simulink model "VCU10"  (R2021b)
settings: Solver=FixedStepDiscrete  StartTime=0.0  StopTime=10.0  FixedStep=0.01  RelTol=1e-3
values from neighbouring files (symbols this model uses):
  F = 0.0    [VCU10DB.sldd]
  FSEC_ESP_EMERGENCY_PRESSURE_MPA = 8.0    [VCU10DB.sldd]
  T = 1.0    [VCU10DB.sldd]
libraries: simulink x148, hdlsllib x90
(part 3 of 4)

== system VCU10/EPS/EPS_ReceiveMsg/EPS_Send_Msg2 ==
  canb_epssendmsg2 : Inport
  Add1 : Sum  Inputs=-++
  Add2 : Sum
  Add5 : Sum  Inputs=-++
  Bit Shift1 : hdlsllib/Logic and Bit Operations/Bit Shift  mode=Shift Left Logical  N=8
  Bus Creator : BusCreator  Inputs=5
  Constant1 : Constant  Value=1024  OutDataTypeStr=uint16
  Constant2 : Constant  Value=1024  OutDataTypeStr=uint16
  Data Type Conversion1 : DataTypeConversion  OutDataTypeStr=double
  Data Type Conversion{3..6,8,10} (6 alike) : DataTypeConversion  OutDataTypeStr=uint16
  Data Type Conversion2 : DataTypeConversion  OutDataTypeStr=double
  Demux : Demux  Outputs=8
  Gain1 : Gain  Gain=256
  Gain2 : Gain  Gain=256
  canb_epssendmsg2signal : Outport
  wires:
  canb_epssendmsg2/1 -> Demux/1
  Bus Creator/1 -> canb_epssendmsg2signal/1
  Demux/1 -> Bus Creator/1  "eps_mode"
  Data Type Conversion2/1 -> Bus Creator/4  "actual_angle"
  Data Type Conversion6/1 -> Gain2/1
  Data Type Conversion5/1 -> Add1/3
  Constant1/1 -> Add1/1
  Gain2/1 -> Add1/2
  Add1/1 -> Data Type Conversion2/1
  Data Type Conversion1/1 -> Bus Creator/3  "received_angle"
  Data Type Conversion8/1 -> Gain1/1
  Data Type Conversion10/1 -> Add5/3
  Constant2/1 -> Add5/1
  Gain1/1 -> Add5/2
  Add5/1 -> Data Type Conversion1/1
  Add2/1 -> Bus Creator/2  "received_command_number"
  Bit Shift1/1 -> Add2/1
  Data Type Conversion3/1 -> Bit Shift1/1
  Data Type Conversion4/1 -> Add2/2
  Demux/2 -> Data Type Conversion3/1  "eps_send_cound"
  Demux/3 -> Data Type Conversion4/1
  Demux/4 -> Data Type Conversion8/1
  Demux/5 -> Data Type Conversion10/1
  Demux/6 -> Data Type Conversion6/1
  Demux/7 -> Data Type Conversion5/1
  Demux/8 -> Bus Creator/5  "eps_send_cound"

== system VCU10/EPS/EPS_TransmitMsg/Subsystem2 ==
  eps_wheel_angle : Inport
  Add1 : Sum
  Constant1 : Constant  Value=1024  OutDataTypeStr=double
  Data Type Conversion4 : DataTypeConversion  OutDataTypeStr=double
  Data Type Conversion5 : DataTypeConversion  OutDataTypeStr=uint32
  Gain1 : Gain  Gain=5
  ipc_cmdangle : Outport
  wires:
  Constant1/1 -> Add1/1
  Add1/1 -> Data Type Conversion5/1
  Data Type Conversion4/1 -> Gain1/1
  Gain1/1 -> Add1/2
  eps_wheel_angle/1 -> Data Type Conversion4/1
  Data Type Conversion5/1 -> ipc_cmdangle/1

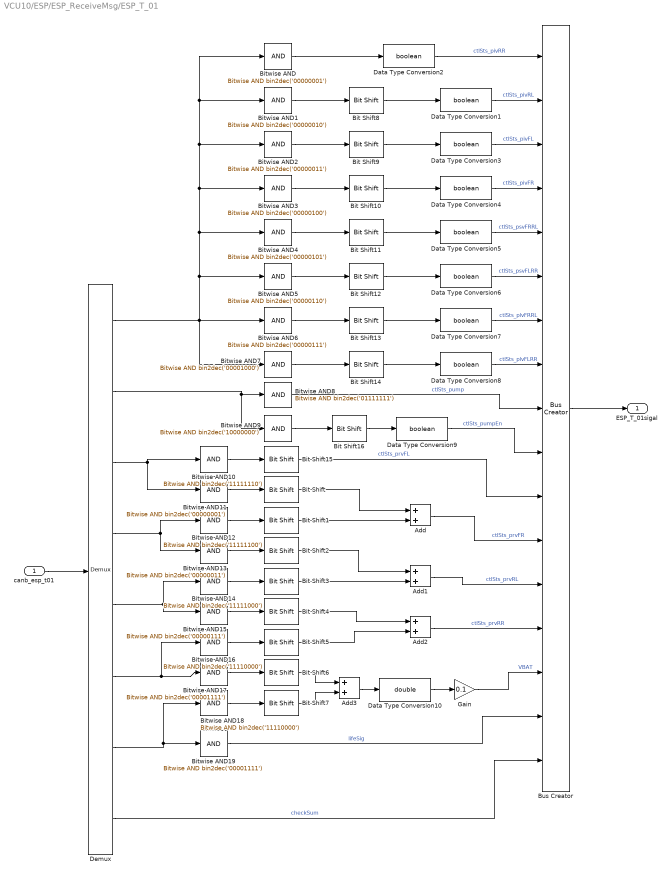
== system VCU10/ESP/ESP_ReceiveMsg/ESP_T_01 ==
  canb_esp_t01 : Inport
  Add{,1..3} (4 alike) : Sum
  Bit Shift : hdlsllib/Logic and Bit Operations/Bit Shift  mode=Shift Left Logical  N=6
  Bit Shift1 : hdlsllib/Logic and Bit Operations/Bit Shift  mode=Shift Right Logical  N=2
  Bit Shift10 : hdlsllib/Logic and Bit Operations/Bit Shift  mode=Shift Right Logical  N=3
  Bit Shift11 : hdlsllib/Logic and Bit Operations/Bit Shift  mode=Shift Right Logical  N=4
  Bit Shift12 : hdlsllib/Logic and Bit Operations/Bit Shift  mode=Shift Right Logical  N=5
  Bit Shift13 : hdlsllib/Logic and Bit Operations/Bit Shift  mode=Shift Right Logical  N=6
  Bit Shift14 : hdlsllib/Logic and Bit Operations/Bit Shift  mode=Shift Right Logical  N=7
  Bit Shift15 : hdlsllib/Logic and Bit Operations/Bit Shift  mode=Shift Right Logical  N=1
  Bit Shift16 : hdlsllib/Logic and Bit Operations/Bit Shift  mode=Shift Right Logical  N=7
  Bit Shift2 : hdlsllib/Logic and Bit Operations/Bit Shift  mode=Shift Left Logical  N=5
  Bit Shift3 : hdlsllib/Logic and Bit Operations/Bit Shift  mode=Shift Right Logical  N=3
  Bit Shift4 : hdlsllib/Logic and Bit Operations/Bit Shift  mode=Shift Left Logical  N=4
  Bit Shift5 : hdlsllib/Logic and Bit Operations/Bit Shift  mode=Shift Right Logical  N=4
  Bit Shift6 : hdlsllib/Logic and Bit Operations/Bit Shift  mode=Shift Left Logical  N=4
  Bit Shift7 : hdlsllib/Logic and Bit Operations/Bit Shift  mode=Shift Right Logical  N=4
  Bit Shift8 : hdlsllib/Logic and Bit Operations/Bit Shift  mode=Shift Right Logical  N=1
  Bit Shift9 : hdlsllib/Logic and Bit Operations/Bit Shift  mode=Shift Right Logical  N=2
  Bitwise AND : simulink/Logic and Bit Operations/Bitwise Operator  logicop=AND  UseBitMask=on  BitMask=bin2dec('00000001')  BitMaskRealWorld=Stored Integer
  Bitwise AND1 : simulink/Logic and Bit Operations/Bitwise Operator  logicop=AND  UseBitMask=on  BitMask=bin2dec('00000010')  BitMaskRealWorld=Stored Integer
  Bitwise AND10 : simulink/Logic and Bit Operations/Bitwise Operator  logicop=AND  UseBitMask=on  BitMask=bin2dec('11111110')  BitMaskRealWorld=Stored Integer
  Bitwise AND11 : simulink/Logic and Bit Operations/Bitwise Operator  logicop=AND  UseBitMask=on  BitMask=bin2dec('00000001')  BitMaskRealWorld=Stored Integer
  Bitwise AND12 : simulink/Logic and Bit Operations/Bitwise Operator  logicop=AND  UseBitMask=on  BitMask=bin2dec('11111100')  BitMaskRealWorld=Stored Integer
  Bitwise AND13 : simulink/Logic and Bit Operations/Bitwise Operator  logicop=AND  UseBitMask=on  BitMask=bin2dec('00000011')  BitMaskRealWorld=Stored Integer
  Bitwise AND14 : simulink/Logic and Bit Operations/Bitwise Operator  logicop=AND  UseBitMask=on  BitMask=bin2dec('11111000')  BitMaskRealWorld=Stored Integer
  Bitwise AND15 : simulink/Logic and Bit Operations/Bitwise Operator  logicop=AND  UseBitMask=on  BitMask=bin2dec('00000111')  BitMaskRealWorld=Stored Integer
  Bitwise AND16 : simulink/Logic and Bit Operations/Bitwise Operator  logicop=AND  UseBitMask=on  BitMask=bin2dec('11110000')  BitMaskRealWorld=Stored Integer
  Bitwise AND17 : simulink/Logic and Bit Operations/Bitwise Operator  logicop=AND  UseBitMask=on  BitMask=bin2dec('00001111')  BitMaskRealWorld=Stored Integer
  Bitwise AND18 : simulink/Logic and Bit Operations/Bitwise Operator  logicop=AND  UseBitMask=on  BitMask=bin2dec('11110000')  BitMaskRealWorld=Stored Integer
  Bitwise AND19 : simulink/Logic and Bit Operations/Bitwise Operator  logicop=AND  UseBitMask=on  BitMask=bin2dec('00001111')  BitMaskRealWorld=Stored Integer
  Bitwise AND2 : simulink/Logic and Bit Operations/Bitwise Operator  logicop=AND  UseBitMask=on  BitMask=bin2dec('00000011')  BitMaskRealWorld=Stored Integer
  Bitwise AND3 : simulink/Logic and Bit Operations/Bitwise Operator  logicop=AND  UseBitMask=on  BitMask=bin2dec('00000100')  BitMaskRealWorld=Stored Integer
  Bitwise AND4 : simulink/Logic and Bit Operations/Bitwise Operator  logicop=AND  UseBitMask=on  BitMask=bin2dec('00000101')  BitMaskRealWorld=Stored Integer
  Bitwise AND5 : simulink/Logic and Bit Operations/Bitwise Operator  logicop=AND  UseBitMask=on  BitMask=bin2dec('00000110')  BitMaskRealWorld=Stored Integer
  Bitwise AND6 : simulink/Logic and Bit Operations/Bitwise Operator  logicop=AND  UseBitMask=on  BitMask=bin2dec('00000111')  BitMaskRealWorld=Stored Integer
  Bitwise AND7 : simulink/Logic and Bit Operations/Bitwise Operator  logicop=AND  UseBitMask=on  BitMask=bin2dec('00001000')  BitMaskRealWorld=Stored Integer
  Bitwise AND8 : simulink/Logic and Bit Operations/Bitwise Operator  logicop=AND  UseBitMask=on  BitMask=bin2dec('01111111')  BitMaskRealWorld=Stored Integer
  Bitwise AND9 : simulink/Logic and Bit Operations/Bitwise Operator  logicop=AND  UseBitMask=on  BitMask=bin2dec('10000000')  BitMaskRealWorld=Stored Integer
  Bus Creator : BusCreator  Inputs=17
  Data Type Conversion{1..9} (9 alike) : DataTypeConversion  OutDataTypeStr=boolean
  Data Type Conversion10 : DataTypeConversion  OutDataTypeStr=double
  Demux : Demux  Outputs=8
  Gain : Gain  Gain=0.1
  ESP_T_01sigal : Outport
  wires:
  canb_esp_t01/1 -> Demux/1
  Bus Creator/1 -> ESP_T_01sigal/1
  Bitwise AND/1 -> Data Type Conversion2/1
  Demux/1 -> Bitwise AND/1, Bitwise AND1/1, Bitwise AND2/1, Bitwise AND3/1, Bitwise AND4/1, Bitwise AND5/1, Bitwise AND7/1, Bitwise AND6/1
  Demux/2 -> Bitwise AND9/1, Bitwise AND8/1
  Bitwise AND8/1 -> Bus Creator/9  "ctlSts_pump"
  Bitwise AND10/1 -> Bit Shift15/1
  Demux/4 -> Bitwise AND12/1, Bitwise AND13/1
  Demux/3 -> Bitwise AND10/1, Bitwise AND11/1
  Bitwise AND11/1 -> Bit Shift/1
  Bitwise AND12/1 -> Bit Shift1/1
  Bit Shift1/1 -> Add/2
  Bit Shift/1 -> Add/1
  Add/1 -> Bus Creator/12  "ctlSts_prvFR"
  Bitwise AND13/1 -> Bit Shift2/1
  Demux/5 -> Bitwise AND14/1, Bitwise AND15/1
  Bitwise AND14/1 -> Bit Shift3/1
  Bit Shift2/1 -> Add1/1
  Bit Shift3/1 -> Add1/2
  Add1/1 -> Bus Creator/13  "ctlSts_prvRL"
  Bitwise AND15/1 -> Bit Shift4/1
  Demux/6 -> Bitwise AND16/1, Bitwise AND17/1
  Bitwise AND16/1 -> Bit Shift5/1
  Bit Shift4/1 -> Add2/1
  Bit Shift5/1 -> Add2/2
  Add2/1 -> Bus Creator/14  "ctlSts_prvRR"
  Bitwise AND17/1 -> Bit Shift6/1
  Demux/7 -> Bitwise AND18/1, Bitwise AND19/1
  Bitwise AND18/1 -> Bit Shift7/1
  Bit Shift6/1 -> Add3/1
  Bit Shift7/1 -> Add3/2
  Bitwise AND19/1 -> Bus Creator/16  "lifeSig"
  Demux/8 -> Bus Creator/17  "checkSum"
  Bitwise AND1/1 -> Bit Shift8/1
  Bit Shift8/1 -> Data Type Conversion1/1
  Bitwise AND2/1 -> Bit Shift9/1
  Bit Shift9/1 -> Data Type Conversion3/1
  Bitwise AND3/1 -> Bit Shift10/1
  Bitwise AND4/1 -> Bit Shift11/1
  Bitwise AND5/1 -> Bit Shift12/1
  Bitwise AND6/1 -> Bit Shift13/1
  Bitwise AND7/1 -> Bit Shift14/1
  Bit Shift10/1 -> Data Type Conversion4/1
  Bit Shift11/1 -> Data Type Conversion5/1
  Bit Shift12/1 -> Data Type Conversion6/1
  Bit Shift13/1 -> Data Type Conversion7/1
  Bit Shift14/1 -> Data Type Conversion8/1
  Gain/1 -> Bus Creator/15  "VBAT"
  Data Type Conversion2/1 -> Bus Creator/1  "ctlSts_pivRR"
  Data Type Conversion1/1 -> Bus Creator/2  "ctlSts_pivRL"
  Data Type Conversion3/1 -> Bus Creator/3  "ctlSts_pivFL"
  Data Type Conversion4/1 -> Bus Creator/4  "ctlSts_pivFR"
  Data Type Conversion5/1 -> Bus Creator/5  "ctlSts_psvFRRL"
  Data Type Conversion6/1 -> Bus Creator/6  "ctlSts_psvFLRR"
  Data Type Conversion7/1 -> Bus Creator/7  "ctlSts_plvFRRL"
  Data Type Conversion8/1 -> Bus Creator/8  "ctlSts_plvFLRR"
  Bit Shift15/1 -> Bus Creator/11  "ctlSts_prvFL"
  Bitwise AND9/1 -> Bit Shift16/1
  Bit Shift16/1 -> Data Type Conversion9/1
  Data Type Conversion9/1 -> Bus Creator/10  "ctlSts_pumpEn"
  Data Type Conversion10/1 -> Gain/1
  Add3/1 -> Data Type Conversion10/1

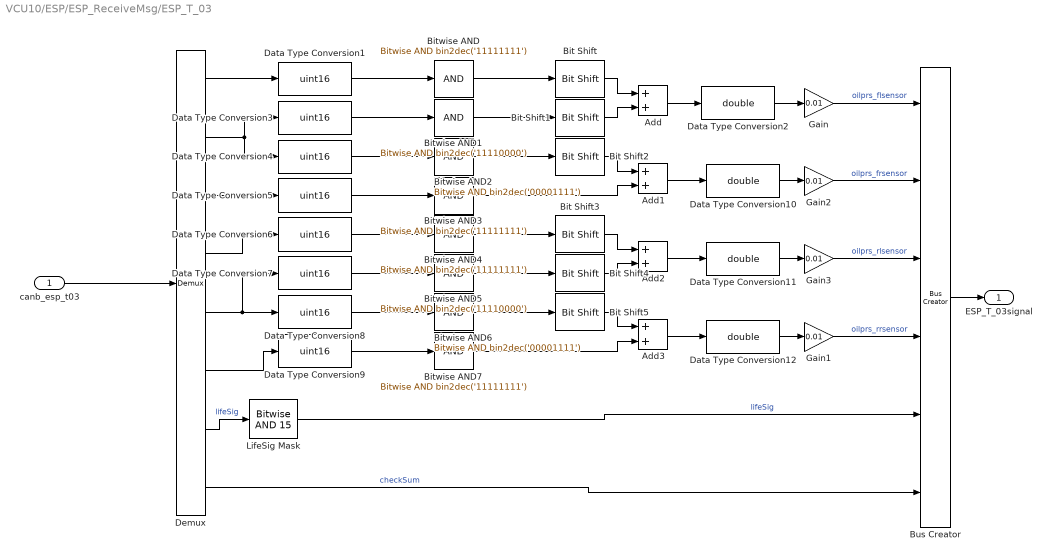
== system VCU10/ESP/ESP_ReceiveMsg/ESP_T_03 ==
  canb_esp_t03 : Inport
  Add{,1..3} (4 alike) : Sum
  Bit Shift : hdlsllib/Logic and Bit Operations/Bit Shift  mode=Shift Left Logical  N=4
  Bit Shift1 : hdlsllib/Logic and Bit Operations/Bit Shift  mode=Shift Right Logical  N=4
  Bit Shift2 : hdlsllib/Logic and Bit Operations/Bit Shift  mode=Shift Left Logical  N=8
  Bit Shift3 : hdlsllib/Logic and Bit Operations/Bit Shift  mode=Shift Left Logical  N=4
  Bit Shift4 : hdlsllib/Logic and Bit Operations/Bit Shift  mode=Shift Right Logical  N=4
  Bit Shift5 : hdlsllib/Logic and Bit Operations/Bit Shift  mode=Shift Left Logical  N=8
  Bitwise AND{,3..4,7} (4 alike) : simulink/Logic and Bit Operations/Bitwise Operator  logicop=AND  UseBitMask=on  BitMask=bin2dec('11111111')  BitMaskRealWorld=Stored Integer
  Bitwise AND1 : simulink/Logic and Bit Operations/Bitwise Operator  logicop=AND  UseBitMask=on  BitMask=bin2dec('11110000')  BitMaskRealWorld=Stored Integer
  Bitwise AND2 : simulink/Logic and Bit Operations/Bitwise Operator  logicop=AND  UseBitMask=on  BitMask=bin2dec('00001111')  BitMaskRealWorld=Stored Integer
  Bitwise AND5 : simulink/Logic and Bit Operations/Bitwise Operator  logicop=AND  UseBitMask=on  BitMask=bin2dec('11110000')  BitMaskRealWorld=Stored Integer
  Bitwise AND6 : simulink/Logic and Bit Operations/Bitwise Operator  logicop=AND  UseBitMask=on  BitMask=bin2dec('00001111')  BitMaskRealWorld=Stored Integer
  Bus Creator : BusCreator  Inputs=6
  Data Type Conversion{1,3..9} (8 alike) : DataTypeConversion  OutDataTypeStr=uint16
  Data Type Conversion{2,10..12} (4 alike) : DataTypeConversion  OutDataTypeStr=double
  Demux : Demux  Outputs=8
  Gain{,1..3} (4 alike) : Gain  Gain=0.01
  LifeSig Mask : simulink/Logic and Bit Operations/Bitwise Operator  logicop=AND  UseBitMask=on  BitMask=15  BitMaskRealWorld=Stored Integer
  ESP_T_03signal : Outport
  wires:
  canb_esp_t03/1 -> Demux/1
  Demux/1 -> Data Type Conversion1/1
  Demux/2 -> Data Type Conversion3/1, Data Type Conversion4/1
  Data Type Conversion1/1 -> Bitwise AND/1
  Data Type Conversion3/1 -> Bitwise AND1/1
  Bitwise AND/1 -> Bit Shift/1
  Bitwise AND1/1 -> Bit Shift1/1
  Bit Shift/1 -> Add/1
  Bit Shift1/1 -> Add/2
  Demux/3 -> Data Type Conversion5/1
  Data Type Conversion4/1 -> Bitwise AND2/1
  Bitwise AND2/1 -> Bit Shift2/1
  Data Type Conversion5/1 -> Bitwise AND3/1
  Bit Shift2/1 -> Add1/1
  Bitwise AND3/1 -> Add1/2
  Data Type Conversion6/1 -> Bitwise AND4/1
  Data Type Conversion7/1 -> Bitwise AND5/1
  Bitwise AND4/1 -> Bit Shift3/1
  Bitwise AND5/1 -> Bit Shift4/1
  Bit Shift3/1 -> Add2/1
  Bit Shift4/1 -> Add2/2
  Data Type Conversion8/1 -> Bitwise AND6/1
  Data Type Conversion9/1 -> Bitwise AND7/1
  Bitwise AND6/1 -> Bit Shift5/1
  Bit Shift5/1 -> Add3/1
  Bitwise AND7/1 -> Add3/2
  Demux/4 -> Data Type Conversion6/1
  Demux/5 -> Data Type Conversion8/1, Data Type Conversion7/1
  Demux/6 -> Data Type Conversion9/1
  Demux/8 -> Bus Creator/6  "checkSum"
  Bus Creator/1 -> ESP_T_03signal/1
  Gain/1 -> Bus Creator/1  "oilprs_flsensor"
  Gain3/1 -> Bus Creator/3  "oilprs_rlsensor"
  Gain2/1 -> Bus Creator/2  "oilprs_frsensor"
  Gain1/1 -> Bus Creator/4  "oilprs_rrsensor"
  Add/1 -> Data Type Conversion2/1
  Data Type Conversion2/1 -> Gain/1
  Add1/1 -> Data Type Conversion10/1
  Data Type Conversion10/1 -> Gain2/1
  Add2/1 -> Data Type Conversion11/1
  Data Type Conversion11/1 -> Gain3/1
  Add3/1 -> Data Type Conversion12/1
  Data Type Conversion12/1 -> Gain1/1
  Demux/7 -> LifeSig Mask/1  "lifeSig"
  LifeSig Mask/1 -> Bus Creator/5  "lifeSig"

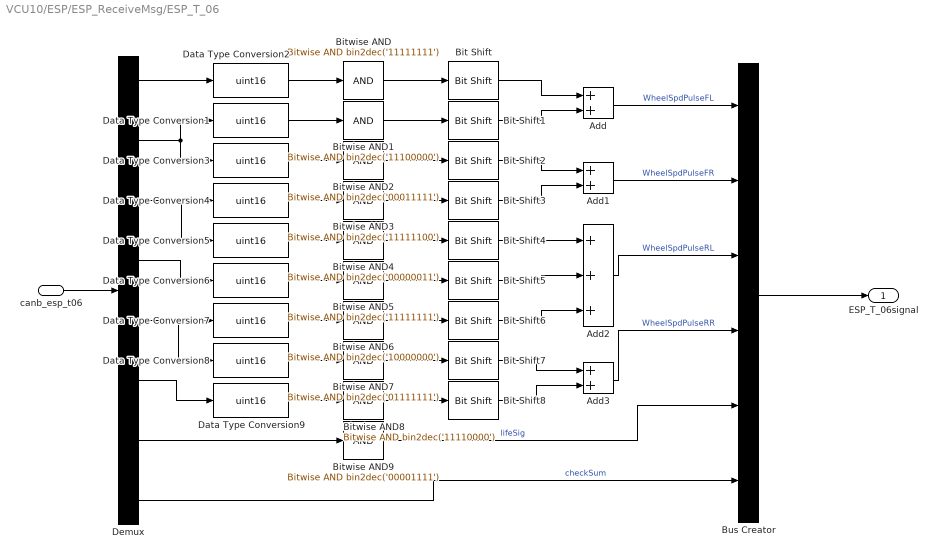
== system VCU10/ESP/ESP_ReceiveMsg/ESP_T_06 ==
  canb_esp_t06 : Inport
  Add : Sum
  Add1 : Sum
  Add2 : Sum  Inputs=+++
  Add3 : Sum
  Bit Shift : hdlsllib/Logic and Bit Operations/Bit Shift  mode=Shift Left Logical  N=3
  Bit Shift1 : hdlsllib/Logic and Bit Operations/Bit Shift  mode=Shift Right Logical  N=5
  Bit Shift2 : hdlsllib/Logic and Bit Operations/Bit Shift  mode=Shift Left Logical  N=6
  Bit Shift3 : hdlsllib/Logic and Bit Operations/Bit Shift  mode=Shift Right Logical  N=2
  Bit Shift4 : hdlsllib/Logic and Bit Operations/Bit Shift  mode=Shift Left Logical  N=9
  Bit Shift5 : hdlsllib/Logic and Bit Operations/Bit Shift  mode=Shift Left Logical  N=1
  Bit Shift6 : hdlsllib/Logic and Bit Operations/Bit Shift  mode=Shift Right Logical  N=7
  Bit Shift7 : hdlsllib/Logic and Bit Operations/Bit Shift  mode=Shift Left Logical  N=4
  Bit Shift8 : hdlsllib/Logic and Bit Operations/Bit Shift  mode=Shift Right Logical  N=4
  Bitwise AND : simulink/Logic and Bit Operations/Bitwise Operator  logicop=AND  UseBitMask=on  BitMask=bin2dec('11111111')  BitMaskRealWorld=Stored Integer
  Bitwise AND1 : simulink/Logic and Bit Operations/Bitwise Operator  logicop=AND  UseBitMask=on  BitMask=bin2dec('11100000')  BitMaskRealWorld=Stored Integer
  Bitwise AND2 : simulink/Logic and Bit Operations/Bitwise Operator  logicop=AND  UseBitMask=on  BitMask=bin2dec('00011111')  BitMaskRealWorld=Stored Integer
  Bitwise AND3 : simulink/Logic and Bit Operations/Bitwise Operator  logicop=AND  UseBitMask=on  BitMask=bin2dec('11111100')  BitMaskRealWorld=Stored Integer
  Bitwise AND4 : simulink/Logic and Bit Operations/Bitwise Operator  logicop=AND  UseBitMask=on  BitMask=bin2dec('00000011')  BitMaskRealWorld=Stored Integer
  Bitwise AND5 : simulink/Logic and Bit Operations/Bitwise Operator  logicop=AND  UseBitMask=on  BitMask=bin2dec('11111111')  BitMaskRealWorld=Stored Integer
  Bitwise AND6 : simulink/Logic and Bit Operations/Bitwise Operator  logicop=AND  UseBitMask=on  BitMask=bin2dec('10000000')  BitMaskRealWorld=Stored Integer
  Bitwise AND7 : simulink/Logic and Bit Operations/Bitwise Operator  logicop=AND  UseBitMask=on  BitMask=bin2dec('01111111')  BitMaskRealWorld=Stored Integer
  Bitwise AND8 : simulink/Logic and Bit Operations/Bitwise Operator  logicop=AND  UseBitMask=on  BitMask=bin2dec('11110000')  BitMaskRealWorld=Stored Integer
  Bitwise AND9 : simulink/Logic and Bit Operations/Bitwise Operator  logicop=AND  UseBitMask=on  BitMask=bin2dec('00001111')  BitMaskRealWorld=Stored Integer
  Bus Creator : BusCreator  Inputs=6
  Data Type Conversion{1..9} (9 alike) : DataTypeConversion  OutDataTypeStr=uint16
  Demux : Demux  Outputs=8
  ESP_T_06signal : Outport
  wires:
  canb_esp_t06/1 -> Demux/1
  Demux/1 -> Data Type Conversion2/1
  Data Type Conversion2/1 -> Bitwise AND/1
  Bitwise AND/1 -> Bit Shift/1
  Data Type Conversion1/1 -> Bitwise AND1/1
  Bitwise AND1/1 -> Bit Shift1/1
  Add/1 -> Bus Creator/1  "WheelSpdPulseFL"
  Bus Creator/1 -> ESP_T_06signal/1
  Demux/2 -> Data Type Conversion3/1, Data Type Conversion1/1
  Data Type Conversion3/1 -> Bitwise AND2/1
  Bitwise AND2/1 -> Bit Shift2/1
  Demux/3 -> Data Type Conversion5/1, Data Type Conversion4/1
  Data Type Conversion4/1 -> Bitwise AND3/1
  Bitwise AND3/1 -> Bit Shift3/1
  Add1/1 -> Bus Creator/2  "WheelSpdPulseFR"
  Bit Shift2/1 -> Add1/1
  Bit Shift3/1 -> Add1/2
  Bit Shift/1 -> Add/1
  Bit Shift1/1 -> Add/2
  Data Type Conversion5/1 -> Bitwise AND4/1
  Bitwise AND4/1 -> Bit Shift4/1
  Demux/4 -> Data Type Conversion6/1
  Data Type Conversion6/1 -> Bitwise AND5/1
  Bitwise AND5/1 -> Bit Shift5/1
  Data Type Conversion7/1 -> Bitwise AND6/1
  Bitwise AND6/1 -> Bit Shift6/1
  Bit Shift4/1 -> Add2/1
  Bit Shift5/1 -> Add2/2
  Bit Shift6/1 -> Add2/3
  Add2/1 -> Bus Creator/3  "WheelSpdPulseRL"
  Demux/5 -> Data Type Conversion8/1, Data Type Conversion7/1
  Data Type Conversion8/1 -> Bitwise AND7/1
  Bitwise AND7/1 -> Bit Shift7/1
  Demux/6 -> Data Type Conversion9/1
  Data Type Conversion9/1 -> Bitwise AND8/1
  Bitwise AND8/1 -> Bit Shift8/1
  Bit Shift7/1 -> Add3/1
  Bit Shift8/1 -> Add3/2
  Add3/1 -> Bus Creator/4  "WheelSpdPulseRR"
  Demux/7 -> Bitwise AND9/1
  Demux/8 -> Bus Creator/6  "checkSum"
  Bitwise AND9/1 -> Bus Creator/5  "lifeSig"

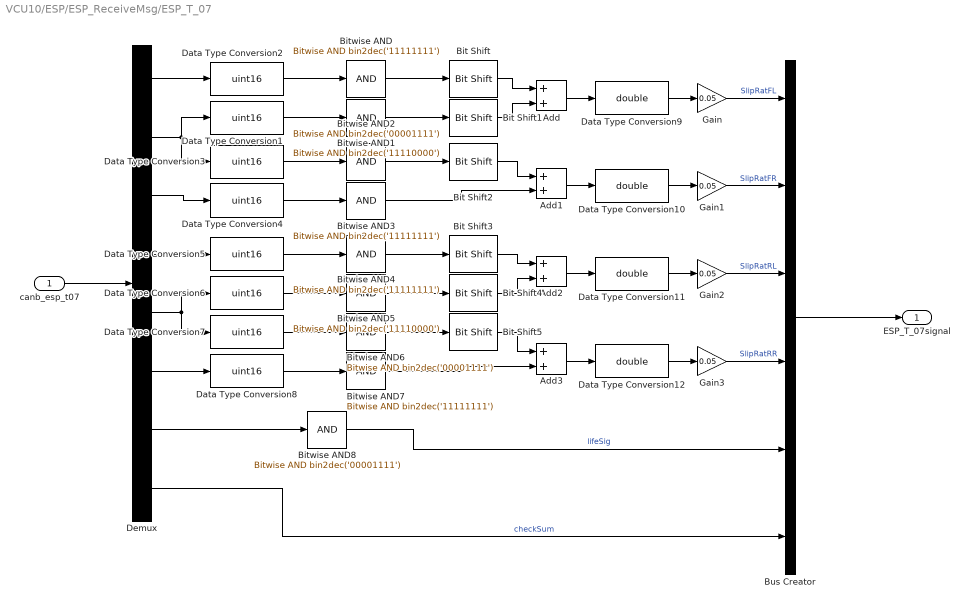
== system VCU10/ESP/ESP_ReceiveMsg/ESP_T_07 ==
  canb_esp_t07 : Inport
  Add{,1..3} (4 alike) : Sum
  Bit Shift : hdlsllib/Logic and Bit Operations/Bit Shift  mode=Shift Left Logical  N=4
  Bit Shift1 : hdlsllib/Logic and Bit Operations/Bit Shift  mode=Shift Right Logical  N=4
  Bit Shift2 : hdlsllib/Logic and Bit Operations/Bit Shift  mode=Shift Left Logical  N=8
  Bit Shift3 : hdlsllib/Logic and Bit Operations/Bit Shift  mode=Shift Left Logical  N=4
  Bit Shift4 : hdlsllib/Logic and Bit Operations/Bit Shift  mode=Shift Right Logical  N=4
  Bit Shift5 : hdlsllib/Logic and Bit Operations/Bit Shift  mode=Shift Left Logical  N=8
  Bitwise AND{,3..4,7} (4 alike) : simulink/Logic and Bit Operations/Bitwise Operator  logicop=AND  UseBitMask=on  BitMask=bin2dec('11111111')  BitMaskRealWorld=Stored Integer
  Bitwise AND1 : simulink/Logic and Bit Operations/Bitwise Operator  logicop=AND  UseBitMask=on  BitMask=bin2dec('11110000')  BitMaskRealWorld=Stored Integer
  Bitwise AND2 : simulink/Logic and Bit Operations/Bitwise Operator  logicop=AND  UseBitMask=on  BitMask=bin2dec('00001111')  BitMaskRealWorld=Stored Integer
  Bitwise AND5 : simulink/Logic and Bit Operations/Bitwise Operator  logicop=AND  UseBitMask=on  BitMask=bin2dec('11110000')  BitMaskRealWorld=Stored Integer
  Bitwise AND6 : simulink/Logic and Bit Operations/Bitwise Operator  logicop=AND  UseBitMask=on  BitMask=bin2dec('00001111')  BitMaskRealWorld=Stored Integer
  Bitwise AND8 : simulink/Logic and Bit Operations/Bitwise Operator  logicop=AND  UseBitMask=on  BitMask=bin2dec('00001111')  BitMaskRealWorld=Stored Integer
  Bus Creator : BusCreator  Inputs=6
  Data Type Conversion{1..8} (8 alike) : DataTypeConversion  OutDataTypeStr=uint16
  Data Type Conversion{9..12} (4 alike) : DataTypeConversion  OutDataTypeStr=double
  Demux : Demux  Outputs=8
  Gain{,1..3} (4 alike) : Gain  Gain=0.05
  ESP_T_07signal : Outport
  wires:
  canb_esp_t07/1 -> Demux/1
  Demux/1 -> Data Type Conversion2/1
  Demux/2 -> Data Type Conversion1/1, Data Type Conversion3/1
  Data Type Conversion1/1 -> Bitwise AND1/1
  Data Type Conversion2/1 -> Bitwise AND/1
  Bitwise AND/1 -> Bit Shift/1
  Bitwise AND1/1 -> Bit Shift1/1
  Bit Shift/1 -> Add/1
  Bit Shift1/1 -> Add/2
  Bus Creator/1 -> ESP_T_07signal/1
  Add/1 -> Data Type Conversion9/1
  Gain/1 -> Bus Creator/1  "SlipRatFL"
  Data Type Conversion3/1 -> Bitwise AND2/1
  Bitwise AND2/1 -> Bit Shift2/1
  Add1/1 -> Data Type Conversion10/1
  Gain1/1 -> Bus Creator/2  "SlipRatFR"
  Bit Shift2/1 -> Add1/1
  Demux/3 -> Data Type Conversion4/1
  Data Type Conversion4/1 -> Bitwise AND3/1
  Bitwise AND3/1 -> Add1/2
  Demux/4 -> Data Type Conversion5/1
  Data Type Conversion5/1 -> Bitwise AND4/1
  Bitwise AND4/1 -> Bit Shift3/1
  Add2/1 -> Data Type Conversion11/1
  Bit Shift3/1 -> Add2/1
  Demux/5 -> Data Type Conversion6/1, Data Type Conversion7/1
  Data Type Conversion6/1 -> Bitwise AND5/1
  Bitwise AND5/1 -> Bit Shift4/1
  Bit Shift4/1 -> Add2/2
  Gain2/1 -> Bus Creator/3  "SlipRatRL"
  Data Type Conversion7/1 -> Bitwise AND6/1
  Bitwise AND6/1 -> Bit Shift5/1
  Demux/6 -> Data Type Conversion8/1
  Data Type Conversion8/1 -> Bitwise AND7/1
  Add3/1 -> Data Type Conversion12/1
  Gain3/1 -> Bus Creator/4  "SlipRatRR"
  Bit Shift5/1 -> Add3/1
  Bitwise AND7/1 -> Add3/2
  Demux/7 -> Bitwise AND8/1
  Demux/8 -> Bus Creator/6  "checkSum"
  Data Type Conversion9/1 -> Gain/1
  Data Type Conversion10/1 -> Gain1/1
  Data Type Conversion11/1 -> Gain2/1
  Data Type Conversion12/1 -> Gain3/1
  Bitwise AND8/1 -> Bus Creator/5  "lifeSig"

== system VCU10/ESP/ESP_ReceiveMsg/Subsystem ==
  lifesig : Inport
  brkmotor_check_system : Stateflow chart  TreatAsAtomicUnit=on
  brkmotor_check : Outport
  wires:
  lifesig/1 -> brkmotor_check_system/1(lifesig)
  brkmotor_check_system/1(brkmotor_check) -> brkmotor_check/1

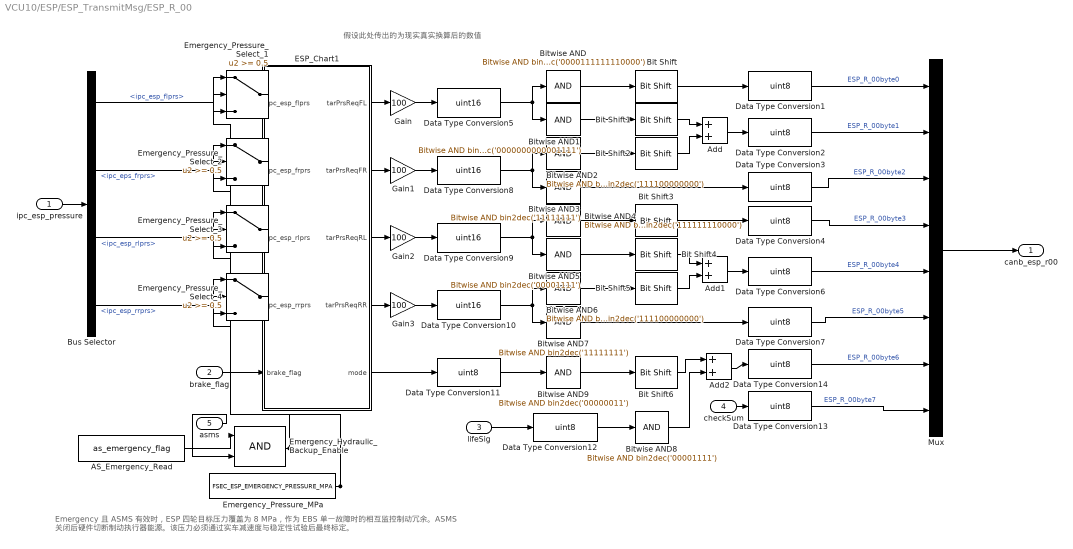
== system VCU10/ESP/ESP_TransmitMsg/ESP_R_00 ==
  note: 假设此处传出的为现实真实换算后的数值
  note: Emergency 且 ASMS 有效时，ESP 四轮目标压力覆盖为 8 MPa，作为 EBS 单一故障时的相互监控制动冗余。ASMS 关闭后硬件切断制动执行器能源。该压力必须通过实车减速度与稳定性试验后最终标定。
  ipc_esp_pressure : Inport
  brake_flag : Inport  Port=2
  lifeSig : Inport  Port=3
  checkSum : Inport  Port=4
  asms : Inport  Port=5  OutDataTypeStr=boolean
  AS_Emergency_Read : DataStoreRead  DataStoreName=as_emergency_flag  IndexOptions=Index vector (dialog)  Indices=1  OutputSizes=1
  Add : Sum
  Add1 : Sum
  Add2 : Sum
  Bit Shift : hdlsllib/Logic and Bit Operations/Bit Shift  mode=Shift Right Logical  N=4
  Bit Shift1 : hdlsllib/Logic and Bit Operations/Bit Shift  mode=Shift Left Logical  N=4
  Bit Shift2 : hdlsllib/Logic and Bit Operations/Bit Shift  mode=Shift Right Logical  N=8
  Bit Shift3 : hdlsllib/Logic and Bit Operations/Bit Shift  mode=Shift Right Logical  N=4
  Bit Shift4 : hdlsllib/Logic and Bit Operations/Bit Shift  mode=Shift Left Logical  N=4
  Bit Shift5 : hdlsllib/Logic and Bit Operations/Bit Shift  mode=Shift Right Logical  N=8
  Bit Shift6 : hdlsllib/Logic and Bit Operations/Bit Shift  mode=Shift Left Logical  N=6
  Bitwise AND : simulink/Logic and Bit Operations/Bitwise Operator  logicop=AND  UseBitMask=on  BitMask=bin2dec('0000111111110000')  BitMaskRealWorld=Stored Integer
  Bitwise AND1 : simulink/Logic and Bit Operations/Bitwise Operator  logicop=AND  UseBitMask=on  BitMask=bin2dec('0000000000001111')  BitMaskRealWorld=Stored Integer
  Bitwise AND2 : simulink/Logic and Bit Operations/Bitwise Operator  logicop=AND  UseBitMask=on  BitMask=bin2dec('111100000000')  BitMaskRealWorld=Stored Integer
  Bitwise AND3 : simulink/Logic and Bit Operations/Bitwise Operator  logicop=AND  UseBitMask=on  BitMask=bin2dec('11111111')  BitMaskRealWorld=Stored Integer
  Bitwise AND4 : simulink/Logic and Bit Operations/Bitwise Operator  logicop=AND  UseBitMask=on  BitMask=bin2dec('111111110000')  BitMaskRealWorld=Stored Integer
  Bitwise AND5 : simulink/Logic and Bit Operations/Bitwise Operator  logicop=AND  UseBitMask=on  BitMask=bin2dec('00001111')  BitMaskRealWorld=Stored Integer
  Bitwise AND6 : simulink/Logic and Bit Operations/Bitwise Operator  logicop=AND  UseBitMask=on  BitMask=bin2dec('111100000000')  BitMaskRealWorld=Stored Integer
  Bitwise AND7 : simulink/Logic and Bit Operations/Bitwise Operator  logicop=AND  UseBitMask=on  BitMask=bin2dec('11111111')  BitMaskRealWorld=Stored Integer
  Bitwise AND8 : simulink/Logic and Bit Operations/Bitwise Operator  logicop=AND  UseBitMask=on  BitMask=bin2dec('00001111')  BitMaskRealWorld=Stored Integer
  Bitwise AND9 : simulink/Logic and Bit Operations/Bitwise Operator  logicop=AND  UseBitMask=on  BitMask=bin2dec('00000011')  BitMaskRealWorld=Stored Integer
  Bus Selector : BusSelector  OutputSignals=ipc_esp_flprs,ipc_eps_frprs,ipc_esp_rlprs,ipc_esp_rrprs
  Data Type Conversion{1..4,6..7,11..14} (10 alike) : DataTypeConversion  OutDataTypeStr=uint8
  Data Type Conversion{5,8..10} (4 alike) : DataTypeConversion  OutDataTypeStr=uint16
  ESP_Chart1 : Stateflow chart  TreatAsAtomicUnit=on
  Emergency_Hydraulic_Backup_Enable : Logic  AllPortsSameDT=off  OutDataTypeStr=boolean
  Emergency_Pressure_MPa : Constant  Value=FSEC_ESP_EMERGENCY_PRESSURE_MPA  OutDataTypeStr=double
  Emergency_Pressure_Select_{1..4} (4 alike) : Switch  Threshold=0.5
  Gain{,1..3} (4 alike) : Gain  Gain=100
  Mux : Mux  Inputs=8
  canb_esp_r00 : Outport
  wires:
  Gain1/1 -> Data Type Conversion8/1
  Bitwise AND7/1 -> Data Type Conversion7/1
  Gain/1 -> Data Type Conversion5/1
  Bit Shift/1 -> Data Type Conversion1/1
  ESP_Chart1/3(tarPrsReqRL) -> Gain2/1
  Add/1 -> Data Type Conversion2/1
  Bitwise AND5/1 -> Bit Shift4/1
  Bitwise AND4/1 -> Bit Shift3/1
  Data Type Conversion1/1 -> Mux/1  "ESP_R_00byte0"
  Data Type Conversion3/1 -> Mux/3  "ESP_R_00byte2"
  brake_flag/1 -> ESP_Chart1/5(brake_flag)
  ESP_Chart1/4(tarPrsReqRR) -> Gain3/1
  Bitwise AND1/1 -> Bit Shift1/1
  Data Type Conversion4/1 -> Mux/4  "ESP_R_00byte3"
  Bit Shift2/1 -> Add/2
  Bitwise AND/1 -> Bit Shift/1
  Bitwise AND2/1 -> Bit Shift2/1
  Gain2/1 -> Data Type Conversion9/1
  Bitwise AND6/1 -> Bit Shift5/1
  Gain3/1 -> Data Type Conversion10/1
  Data Type Conversion6/1 -> Mux/5  "ESP_R_00byte4"
  Data Type Conversion2/1 -> Mux/2  "ESP_R_00byte1"
  ESP_Chart1/2(tarPrsReqFR) -> Gain1/1
  Bit Shift5/1 -> Add1/2
  Bit Shift6/1 -> Add2/1
  Bit Shift4/1 -> Add1/1
  lifeSig/1 -> Data Type Conversion12/1
  ESP_Chart1/5(mode) -> Data Type Conversion11/1
  Bit Shift3/1 -> Data Type Conversion4/1
  Bitwise AND3/1 -> Data Type Conversion3/1
  checkSum/1 -> Data Type Conversion13/1
  Add2/1 -> Data Type Conversion14/1
  Data Type Conversion7/1 -> Mux/6  "ESP_R_00byte5"
  Bitwise AND8/1 -> Add2/2
  Add1/1 -> Data Type Conversion6/1
  ESP_Chart1/1(tarPrsReqFL) -> Gain/1
  Bit Shift1/1 -> Add/1
  Data Type Conversion5/1 -> Bitwise AND1/1, Bitwise AND/1
  Data Type Conversion8/1 -> Bitwise AND3/1, Bitwise AND2/1
  Data Type Conversion9/1 -> Bitwise AND5/1, Bitwise AND4/1
  Data Type Conversion10/1 -> Bitwise AND6/1, Bitwise AND7/1
  Data Type Conversion11/1 -> Bitwise AND9/1
  Data Type Conversion12/1 -> Bitwise AND8/1
  Data Type Conversion13/1 -> Mux/8  "ESP_R_00byte7"
  Bitwise AND9/1 -> Bit Shift6/1
  ipc_esp_pressure/1 -> Bus Selector/1
  Data Type Conversion14/1 -> Mux/7  "ESP_R_00byte6"
  Mux/1 -> canb_esp_r00/1
  AS_Emergency_Read/1 -> Emergency_Hydraulic_Backup_Enable/1
  asms/1 -> Emergency_Hydraulic_Backup_Enable/2
  Emergency_Pressure_MPa/1 -> Emergency_Pressure_Select_1/1, Emergency_Pressure_Select_2/1, Emergency_Pressure_Select_3/1, Emergency_Pressure_Select_4/1
  Emergency_Hydraulic_Backup_Enable/1 -> Emergency_Pressure_Select_1/2, Emergency_Pressure_Select_2/2, Emergency_Pressure_Select_3/2, Emergency_Pressure_Select_4/2
  Bus Selector/1 -> Emergency_Pressure_Select_1/3  "<ipc_esp_flprs>"
  Emergency_Pressure_Select_1/1 -> ESP_Chart1/1(ipc_esp_flprs)
  Bus Selector/2 -> Emergency_Pressure_Select_2/3  "<ipc_eps_frprs>"
  Emergency_Pressure_Select_2/1 -> ESP_Chart1/2(ipc_esp_frprs)
  Bus Selector/3 -> Emergency_Pressure_Select_3/3  "<ipc_esp_rlprs>"
  Emergency_Pressure_Select_3/1 -> ESP_Chart1/3(ipc_esp_rlprs)
  Bus Selector/4 -> Emergency_Pressure_Select_4/3  "<ipc_esp_rrprs>"
  Emergency_Pressure_Select_4/1 -> ESP_Chart1/4(ipc_esp_rrprs)

== system VCU10/IPC/IPC_ReceiveMsg/IPC_Rx_Msg ==
  steer_return : Inport
  ipc_resgo : Inport  Port=2
  ipc_resstop : Inport  Port=3
  ipc_astask : Inport  Port=4
  Add : Sum  Inputs=+++
  Bit Shift : hdlsllib/Logic and Bit Operations/Bit Shift  mode=Shift Left Logical  N=1
  Bit Shift1 : hdlsllib/Logic and Bit Operations/Bit Shift  mode=Shift Left Logical  N=2
  Bitwise AND : simulink/Logic and Bit Operations/Bitwise Operator  logicop=AND  UseBitMask=on  BitMask=bin2dec('00000001')  BitMaskRealWorld=Stored Integer
  Bitwise AND1 : simulink/Logic and Bit Operations/Bitwise Operator  logicop=AND  UseBitMask=on  BitMask=bin2dec('00000001')  BitMaskRealWorld=Stored Integer
  Bitwise AND2 : simulink/Logic and Bit Operations/Bitwise Operator  logicop=AND  UseBitMask=on  BitMask=bin2dec('00000001')  BitMaskRealWorld=Stored Integer
  Data Type Conversion{1..4} (4 alike) : DataTypeConversion  OutDataTypeStr=uint8
  Ground : Ground
  Mux : Mux  Inputs=8
  canb_ipcrxmsg : Outport
  wires:
  Mux/1 -> canb_ipcrxmsg/1
  Ground/1 -> Mux/6, Mux/7, Mux/8, Mux/4, Mux/3, Mux/5
  Data Type Conversion1/1 -> Bitwise AND/1
  Data Type Conversion2/1 -> Bitwise AND1/1
  Bitwise AND/1 -> Add/1
  Bit Shift/1 -> Add/2
  Add/1 -> Mux/1  "canb_ipcrxmsgbyte0"
  Bitwise AND1/1 -> Bit Shift/1
  Data Type Conversion3/1 -> Mux/2  "canb_ipcrxmsgbyte1"
  Data Type Conversion4/1 -> Bitwise AND2/1
  Bitwise AND2/1 -> Bit Shift1/1
  steer_return/1 -> Data Type Conversion1/1
  ipc_resgo/1 -> Data Type Conversion2/1
  ipc_resstop/1 -> Data Type Conversion4/1
  ipc_astask/1 -> Data Type Conversion3/1
  Bit Shift1/1 -> Add/3

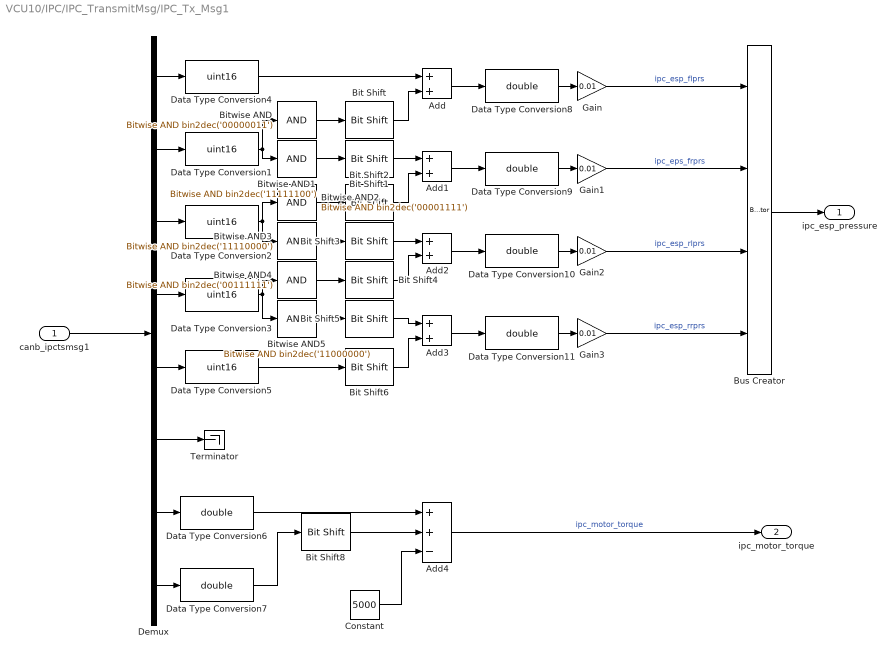
== system VCU10/IPC/IPC_TransmitMsg/IPC_Tx_Msg1 ==
  canb_ipctsmsg1 : Inport
  Add{,1..3} (4 alike) : Sum
  Add4 : Sum  Inputs=++-
  Bit Shift : hdlsllib/Logic and Bit Operations/Bit Shift  mode=Shift Left Logical  N=8
  Bit Shift1 : hdlsllib/Logic and Bit Operations/Bit Shift  mode=Shift Right Logical  N=2
  Bit Shift2 : hdlsllib/Logic and Bit Operations/Bit Shift  mode=Shift Left Logical  N=6
  Bit Shift3 : hdlsllib/Logic and Bit Operations/Bit Shift  mode=Shift Right Logical  N=4
  Bit Shift4 : hdlsllib/Logic and Bit Operations/Bit Shift  mode=Shift Left Logical  N=4
  Bit Shift5 : hdlsllib/Logic and Bit Operations/Bit Shift  mode=Shift Right Logical  N=6
  Bit Shift6 : hdlsllib/Logic and Bit Operations/Bit Shift  mode=Shift Left Logical  N=2
  Bit Shift8 : hdlsllib/Logic and Bit Operations/Bit Shift  mode=Shift Left Logical  N=8
  Bitwise AND : simulink/Logic and Bit Operations/Bitwise Operator  logicop=AND  UseBitMask=on  BitMask=bin2dec('00000011')  BitMaskRealWorld=Stored Integer
  Bitwise AND1 : simulink/Logic and Bit Operations/Bitwise Operator  logicop=AND  UseBitMask=on  BitMask=bin2dec('11111100')  BitMaskRealWorld=Stored Integer
  Bitwise AND2 : simulink/Logic and Bit Operations/Bitwise Operator  logicop=AND  UseBitMask=on  BitMask=bin2dec('00001111')  BitMaskRealWorld=Stored Integer
  Bitwise AND3 : simulink/Logic and Bit Operations/Bitwise Operator  logicop=AND  UseBitMask=on  BitMask=bin2dec('11110000')  BitMaskRealWorld=Stored Integer
  Bitwise AND4 : simulink/Logic and Bit Operations/Bitwise Operator  logicop=AND  UseBitMask=on  BitMask=bin2dec('00111111')  BitMaskRealWorld=Stored Integer
  Bitwise AND5 : simulink/Logic and Bit Operations/Bitwise Operator  logicop=AND  UseBitMask=on  BitMask=bin2dec('11000000')  BitMaskRealWorld=Stored Integer
  Bus Creator : BusCreator  Inputs=4
  Constant : Constant  Value=5000  OutDataTypeStr=uint16
  Data Type Conversion{1..5} (5 alike) : DataTypeConversion  OutDataTypeStr=uint16
  Data Type Conversion{6..11} (6 alike) : DataTypeConversion  OutDataTypeStr=double
  Demux : Demux  Outputs=8
  Gain{,1..3} (4 alike) : Gain  Gain=0.01
  Terminator : Terminator
  ipc_esp_pressure : Outport
  ipc_motor_torque : Outport  Port=2
  wires:
  canb_ipctsmsg1/1 -> Demux/1
  Demux/1 -> Data Type Conversion4/1
  Data Type Conversion1/1 -> Bitwise AND/1, Bitwise AND1/1
  Demux/2 -> Data Type Conversion1/1
  Bitwise AND/1 -> Bit Shift/1
  Data Type Conversion4/1 -> Add/1
  Bit Shift/1 -> Add/2
  Bitwise AND1/1 -> Bit Shift1/1
  Demux/3 -> Data Type Conversion2/1
  Data Type Conversion2/1 -> Bitwise AND2/1, Bitwise AND3/1
  Bitwise AND2/1 -> Bit Shift2/1
  Bit Shift1/1 -> Add1/1
  Bit Shift2/1 -> Add1/2
  Demux/4 -> Data Type Conversion3/1
  Bitwise AND3/1 -> Bit Shift3/1
  Data Type Conversion3/1 -> Bitwise AND5/1, Bitwise AND4/1
  Bitwise AND4/1 -> Bit Shift4/1
  Bit Shift4/1 -> Add2/2
  Bit Shift3/1 -> Add2/1
  Bitwise AND5/1 -> Bit Shift5/1
  Demux/5 -> Data Type Conversion5/1
  Data Type Conversion5/1 -> Bit Shift6/1
  Bit Shift5/1 -> Add3/1
  Bit Shift6/1 -> Add3/2
  Demux/6 -> Terminator/1
  Demux/7 -> Data Type Conversion6/1
  Demux/8 -> Data Type Conversion7/1
  Data Type Conversion7/1 -> Bit Shift8/1
  Data Type Conversion6/1 -> Add4/1
  Bit Shift8/1 -> Add4/2
  Bus Creator/1 -> ipc_esp_pressure/1
  Add4/1 -> ipc_motor_torque/1  "ipc_motor_torque"
  Constant/1 -> Add4/3
  Data Type Conversion8/1 -> Gain/1
  Gain/1 -> Bus Creator/1  "ipc_esp_flprs"
  Add/1 -> Data Type Conversion8/1
  Data Type Conversion9/1 -> Gain1/1
  Gain1/1 -> Bus Creator/2  "ipc_eps_frprs"
  Add1/1 -> Data Type Conversion9/1
  Data Type Conversion10/1 -> Gain2/1
  Gain2/1 -> Bus Creator/3  "ipc_esp_rlprs"
  Add2/1 -> Data Type Conversion10/1
  Data Type Conversion11/1 -> Gain3/1
  Gain3/1 -> Bus Creator/4  "ipc_esp_rrprs"
  Add3/1 -> Data Type Conversion11/1

== system VCU10/IPC/IPC_TransmitMsg/IPC_Tx_Msg2 ==
  canb_ipctsmsg2 : Inport
  Add : Sum  Inputs=++-
  Add1 : Sum
  Add2 : Sum
  Bit Shift : hdlsllib/Logic and Bit Operations/Bit Shift  mode=Shift Left Logical  N=8
  Bit Shift1 : hdlsllib/Logic and Bit Operations/Bit Shift  mode=Shift Right Logical  N=7
  Bit Shift2 : hdlsllib/Logic and Bit Operations/Bit Shift  mode=Shift Right Logical  N=6
  Bit Shift3 : hdlsllib/Logic and Bit Operations/Bit Shift  mode=Shift Right Logical  N=2
  Bit Shift4 : hdlsllib/Logic and Bit Operations/Bit Shift  mode=Shift Left Logical  N=8
  Bit Shift5 : hdlsllib/Logic and Bit Operations/Bit Shift  mode=Shift Left Logical  N=8
  Bitwise AND : simulink/Logic and Bit Operations/Bitwise Operator  logicop=AND  UseBitMask=on  BitMask=bin2dec('10000000')  BitMaskRealWorld=Stored Integer
  Bitwise AND1 : simulink/Logic and Bit Operations/Bitwise Operator  logicop=AND  UseBitMask=on  BitMask=bin2dec('01000000')  BitMaskRealWorld=Stored Integer
  Bitwise AND2 : simulink/Logic and Bit Operations/Bitwise Operator  logicop=AND  UseBitMask=on  BitMask=bin2dec('00111100')  BitMaskRealWorld=Stored Integer
  Constant : Constant  Value=1024  OutDataTypeStr=double
  Data Type Conversion1 : DataTypeConversion  OutDataTypeStr=double
  Data Type Conversion2 : DataTypeConversion  OutDataTypeStr=double
  Data Type Conversion3 : DataTypeConversion  OutDataTypeStr=boolean
  Data Type Conversion4 : DataTypeConversion  OutDataTypeStr=boolean
  Data Type Conversion5 : DataTypeConversion  OutDataTypeStr=uint8
  Data Type Conversion{6..9} (4 alike) : DataTypeConversion  OutDataTypeStr=uint16
  Demux : Demux  Outputs=8
  ipc_eps_angle : Outport
  ipc_eps_velocity : Outport  Port=2
  ipc_err : Outport  Port=3
  task_finish : Outport  Port=4
  ipc_heartbeat : Outport  Port=5
  ipc_lspd : Outport  Port=6
  ipc_hspd : Outport  Port=7
  wires:
  Add1/1 -> ipc_lspd/1
  Bit Shift3/1 -> Data Type Conversion5/1
  Demux/3 -> ipc_eps_velocity/1
  Bit Shift4/1 -> Add1/1
  Constant/1 -> Add/3
  Demux/8 -> Data Type Conversion9/1
  Data Type Conversion2/1 -> Bit Shift/1
  Data Type Conversion7/1 -> Add1/2
  Bitwise AND2/1 -> Bit Shift3/1
  Data Type Conversion8/1 -> Bit Shift5/1
  Data Type Conversion9/1 -> Add2/2
  Demux/1 -> Data Type Conversion2/1
  Bit Shift5/1 -> Add2/1
  Add2/1 -> ipc_hspd/1
  Bit Shift1/1 -> Data Type Conversion3/1
  Demux/5 -> Data Type Conversion6/1
  Data Type Conversion6/1 -> Bit Shift4/1
  Data Type Conversion5/1 -> ipc_heartbeat/1
  Demux/6 -> Data Type Conversion7/1
  Data Type Conversion4/1 -> task_finish/1
  Bit Shift2/1 -> Data Type Conversion4/1
  Demux/4 -> Bitwise AND2/1, Bitwise AND/1, Bitwise AND1/1
  Data Type Conversion3/1 -> ipc_err/1
  Add/1 -> ipc_eps_angle/1
  Bitwise AND/1 -> Bit Shift1/1
  Bitwise AND1/1 -> Bit Shift2/1
  canb_ipctsmsg2/1 -> Demux/1
  Demux/2 -> Data Type Conversion1/1
  Bit Shift/1 -> Add/1
  Data Type Conversion1/1 -> Add/2
  Demux/7 -> Data Type Conversion8/1

== system VCU10/LED_Control/EBS_LED/Enabled Subsystem ==
  In1 : Inport
  Enable : EnablePort
  Out1 : Outport
  wires:
  In1/1 -> Out1/1

== system VCU10/Res/Res_Msg/Subsystem ==
  note: 异或校验可靠性判断
  note: 赛车端与VCU断联
  note: 赛车端与遥控端断联
  res_communication : Inport
  res_heartbeat : Inport  Port=2
  res_xorcheck : Inport  Port=3
  xor_consequence : Inport  Port=4
  Logical Operator : Logic  Inputs=3  AllPortsSameDT=off  OutDataTypeStr=boolean
  heaartbeat_chart : Stateflow chart  TreatAsAtomicUnit=on
  xor_Check : Stateflow chart  TreatAsAtomicUnit=on
  res_check : Outport
  wires:
  res_heartbeat/1 -> heaartbeat_chart/1(res_heartbeat)
  heaartbeat_chart/1(res_hbcheck) -> Logical Operator/2
  res_communication/1 -> Logical Operator/1
  Logical Operator/1 -> res_check/1
  res_xorcheck/1 -> xor_Check/1(res_xorcheck)
  xor_consequence/1 -> xor_Check/2(xor_consequence)
  xor_Check/1(xorcheck) -> Logical Operator/3

== stateflow chart VCU10/AS_Stateflow/Chart ==
  state AS_Driving
    state R2D
      en:
      r2d_flag=1;
      as_ready_flag=0;
      as_driving_flag=1;
    state go
      ts_flag=1;
      r2d_flag=0;
      steering_flag=1;
      brake_flag=1;
      ebs_system_flag=1;
      as_led_yellow=2;
      as_led_blue=0;
      as_off_flag=0;
      as_ready_flag=0;
      as_driving_flag=1;
      as_finished_flag=0;
      as_emergency_flag=0;
      manual_driving_flag=0;
    (default) -> R2D
    R2D -> go : [steer_zero==1]
        | {steer_return=F;r2d_warning=F}
  state AS_Ready
    ts_flag=1;
    r2d_flag=0;
    steering_flag=1;
    brake_flag=2;
    ebs_system_flag=1;
    as_led_yellow=1;
    as_led_blue=0;
    as_off_flag=0;
    as_ready_flag=1;
    as_driving_flag=0;
    as_finished_flag=0;
    as_emergency_flag=0;
    manual_driving_flag=0;
    as_ebs_trig=0;
  state transition
  state AS_Off
    ts_flag=0;
    r2d_flag=0;
    steering_flag=0;
    brake_flag=0;
    ebs_system_flag=0;
    as_led_yellow=0;
    as_led_blue=0;
    as_off_flag=1;
    as_ready_flag=0;
    as_driving_flag=0;
    as_finished_flag=0;
    as_emergency_flag=0;
    manual_driving_flag=0;
    as_ebs_trig=0;
  state AS_Emergency
    ts_flag=0;
    r2d_flag=0;
    steering_flag=1;
    brake_flag=1;
    ebs_system_flag=2;
    as_ebs_trig=1;
    as_led_yellow=0;
    as_led_blue=2;
    as_off_flag=0;
    as_ready_flag=0;
    as_driving_flag=0;
    as_finished_flag=0;
    as_emergency_flag=1;
    manual_driving_flag=0;
    safety_lock=1;
  state AS_Finished
    ts_flag=0;
    r2d_flag=0;
    steering_flag=0;
    brake_flag=0;
    ebs_system_flag=2;
    as_ebs_trig=1;
    as_led_yellow=0;
    as_led_blue=1;
    as_off_flag=0;
    as_ready_flag=0;
    as_driving_flag=0;
    as_finished_flag=1;
    as_emergency_flag=0;
    manual_driving_flag=0;
    safety_lock=1;
  state Manual_Driving
    ts_flag=0;
    r2d_flag=0;
    steering_flag=0;
    brake_flag=0;
    ebs_system_flag=0;
    as_led_yellow=0;
    as_led_blue=0;
    as_off_flag=0;
    as_ready_flag=0;
    as_driving_flag=0;
    as_finished_flag=0;
    as_emergency_flag=0;
    manual_driving_flag=1;
    as_ebs_trig=0;
  AS_Driving -> AS_Finished [order 2] : [car_spdzero==1&&task_finish==1&&safety_fault==0&&asms_button==1&&res_stop==0]{as_ebs_trig=1}
  AS_Ready -> (junction 54) [order 2] : after(5,sec)
  (junction 54) -> AS_Driving [order 2] : [res_go==1&&safety_fault==0&&asms_button==1&&res_stop==0]{r2d_warning=T;steer_return=T}
  (junction 54) -> AS_Emergency [order 1] : [ebs_working==1||safety_fault==1||asms_button==0||res_stop==1]
  (junction 53) -> AS_Ready [order 2] : [asb_check==1&&safety_fault==0&&safety_lock==0]
  AS_Driving -> (junction 136) [order 3] : [ami_inspection==1]
  AS_Ready -> AS_Emergency [order 1] : [ebs_working==1||safety_fault==1||asms_button==0||res_stop==1]
  AS_Driving -> AS_Emergency [order 1] : [ebs_working==1||safety_fault==1||asms_button==0||res_stop==1]
  (junction 53) -> AS_Emergency [order 1] : [ebs_working==1||safety_fault==1||asms_button==0||res_stop==1]
  transition -> (junction 53) [order 1] : [ts==1]
  (junction 136) -> AS_Emergency [order 1] : [ebs_working==1||safety_fault==1||asms_button==0||res_stop==1]
  (junction 136) -> AS_Finished [order 2] : after(27,sec)[safety_fault==0&&asms_button==1&&res_stop==0]{as_ebs_trig=1}
  transition -> AS_Emergency [order 2] : [ebs_working==1||safety_fault==1||asms_button==0||res_stop==1]
  AS_Off -> transition [order 2] : [as_task==1&&asms_button==1&&safety_fault==0&&safety_lock==0]{brake_flag=2}
  (default) -> AS_Off
  (junction 55) -> AS_Off : [asms_button==0&&brake_on==0]
  AS_Finished -> AS_Emergency : [res_stop==1]
  AS_Off -> (junction 56) [order 1] : [ami_manualdriving==1&&safety_fault==0&&safety_lock==0]
  (junction 56) -> AS_Off [order 2]
  (junction 57) -> AS_Off [order 2]
  Manual_Driving -> AS_Off : [ts==0]
  (junction 56) -> (junction 57) [order 1] : [ebs_check==0]
  (junction 57) -> Manual_Driving [order 1] : [ts==1]
  data: asms_button input; ebs_check input; ami_manualdriving input; as_task input; ts input; ebs_warning input; ebs_working input; brake_on input; asb_check input; car_spdzero input; task_finish input; res_go input; steer_zero input; safety_fault input boolean; res_stop input; as_ebs_trig output; r2d_warning output; as_led_blue output; as_led_yellow output; steer_return output; steering_flag output; safety_lock output double =0; brake_flag output; manual_driving_flag output; as_emergency_flag output; ebs_system_flag output; as_off_flag output; as_ready_flag output; as_driving_flag output; as_finished_flag output; r2d_flag output; ts_flag output; T parameter; F parameter; ami_inspection input

== stateflow chart VCU10/LED_Control/TSLED_Inspection ==
  state Inspection
    en:
    led_imderr=T;
    led_bmserr=T;
  state Normal
    en:
    led_imderr=F;
    led_bmserr=F;
  (default) -> Inspection
  Inspection -> Normal : [after(2,sec)]
  data: led_imderr output boolean; led_bmserr output boolean; T parameter; F parameter

== stateflow chart VCU10/TS_Activation/Chart ==
  state Ignition_Check
    state begin
      di8_flag=F;
    state DI8_Check_Flag
      (default) -> (junction 5)
      (junction 5) -> (junction 7) [order 1] : [di8_button==0]
      (junction 5) -> (junction 9) [order 2] : {di8_check_flag=0;}
      (junction 7) -> (junction 8) : {di8_check_flag=1;}
      (junction 8) -> (junction 9)
      (junction 9) -> (junction 10)
    state Check
      (default) -> (junction 23)
      (junction 23) -> (junction 25) [order 1] : [di8_button==1]
      (junction 23) -> (junction 29) [order 2]
      (junction 25) -> (junction 27) : {di8_flag=T;di8=T;}
      (junction 27) -> (junction 29)
      (junction 29) -> (junction 32)
    (default) -> begin
    begin -> DI8_Check_Flag
    (junction 17) -> DI8_Check_Flag [order 1] : [di8_check_flag==0]
    Check -> (junction 17)
    (junction 17) -> Check [order 2] : [di8_check_flag==1]
    DI8_Check_Flag -> (junction 17)
  state Flameout_Check
    state DI8_Offcheck_Flag
      (default) -> (junction 39)
      (junction 39) -> (junction 42) [order 1] : [di8_button==0]
      (junction 42) -> (junction 44) : {di8_offcheck_flag=1;}
      (junction 39) -> (junction 46) [order 2] : {di8_offcheck_flag}
      (junction 44) -> (junction 46)
      (junction 46) -> (junction 49)
    state Checkoff
      (default) -> (junction 63)
      (junction 63) -> (junction 61) [order 1] : [di8_button==1]
      (junction 63) -> (junction 57) [order 2]
      (junction 61) -> (junction 60) : {di8_flag=F;di8=F;}
      (junction 60) -> (junction 57)
      (junction 57) -> (junction 58)
    (default) -> DI8_Offcheck_Flag
    (junction 52) -> DI8_Offcheck_Flag [order 1] : [di8_offcheck_flag==0]
    (junction 52) -> Checkoff [order 3]
    (junction 52) -> Checkoff [order 2] : [di8_offcheck_flag==1]
    DI8_Offcheck_Flag -> (junction 52)
  (default) -> Ignition_Check
  Ignition_Check -> Flameout_Check : [di8_flag==T]
  Flameout_Check -> Ignition_Check : [di8_flag==F]
  data: di8_button input; di8 output boolean; di8_offcheck_flag local =0; di8_check_flag local =0; T parameter; F parameter; di8_flag local =F

== stateflow chart VCU10/Motor_Control/Motor_Torque_Stateflow ==
  state Default
    en:
    motor_torque=0;
    du:
    motor_torque=0;
  state AS_Driving
    en:
    motor_torque=as_torque;
    du:
    motor_torque=as_torque;
  state Manual_Driving
    en:
    motor_torque=manual_torque;
    du:
    motor_torque=manual_torque;
  (default) -> Default
  Default -> AS_Driving [order 2] : [as_task==1]
  AS_Driving -> Default : [as_task==0]
  Default -> Manual_Driving [order 1] : [manual_driving_flag==1]
  Manual_Driving -> Default : [manual_driving_flag==0]
  data: manual_driving_flag input; as_task input; manual_torque input; as_torque input; motor_torque output

== matlab function VCU10/DBC_Debug_Select ==
  data: hin_hw input; hin_sel output; ain_hw input; wheel_f_hw input; wheel_h_hw input; control input; pedal_adc input; air_wheel input; digital input; rx_count input; ain_sel output; wheel_f_sel output; wheel_h_sel output; status_base output; pedal_echo output; air_wheel_echo output
function [hin_sel, ain_sel, wheel_f_sel, wheel_h_sel, status_base, pedal_echo, air_wheel_echo] = dbg_select(hin_hw, ain_hw, wheel_f_hw, wheel_h_hw, control, pedal_adc, air_wheel, digital, rx_count)
%#codegen
% Bench-only CAN override. Any stale control/data frame restores hardware input.
persistent last_count ages initialized
if isempty(initialized)
    last_count = uint8(zeros(4,1));
    ages = repmat(uint8(50),4,1);
    initialized = true;
end
for i = 1:4
    if rx_count(i) ~= last_count(i)
        last_count(i) = rx_count(i);
        ages(i) = uint8(0);
    elseif ages(i) < uint8(50)
        ages(i) = ages(i) + uint8(1);
    end
end
requested = uint8(0);
if control(1) == uint8(165) && control(2) == uint8(90) && ages(1) < uint8(50)
    requested = bitand(control(3), uint8(15));
end
active = uint8(0);
if bitand(requested,uint8(1)) ~= uint8(0)
    active = bitor(active,uint8(1));
    if bitand(requested,uint8(2)) ~= uint8(0) && ages(2) < uint8(50)
        active = bitor(active,uint8(2));
    end
    if bitand(requested,uint8(4)) ~= uint8(0) && ages(3) < uint8(50)
        active = bitor(active,uint8(4));
    end
    if bitand(requested,uint8(8)) ~= uint8(0) && ages(4) < uint8(50)
        active = bitor(active,uint8(8));
    end
end
hin_sel = uint16(hin_hw);
ain_sel = uint16(ain_hw);
wheel_f_sel = single(wheel_f_hw);
wheel_h_sel = single(wheel_h_hw);
if bitand(active,uint8(8)) ~= uint8(0)
    hin_sel = uint16(digital(1)) + bitshift(uint16(digital(2)),8);
end
if bitand(active,uint8(2)) ~= uint8(0)
    ain_sel(1) = uint16(pedal_adc(1)) + bitshift(uint16(pedal_adc(2)),8);
    ain_sel(2) = uint16(pedal_adc(3)) + bitshift(uint16(pedal_adc(4)),8);
    ain_sel(3) = uint16(pedal_adc(5)) + bitshift(uint16(pedal_adc(6)),8);
end
if bitand(active,uint8(4)) ~= uint8(0)
    ain_sel(4) = uint16(air_wheel(1)) + bitshift(uint16(air_wheel(2)),8);
    ain_sel(5) = uint16(air_wheel(3)) + bitshift(uint16(air_wheel(4)),8);
    wheel_f_sel = single(uint16(air_wheel(5)) + bitshift(uint16(air_wheel(6)),8)) * single(0.1);
    wheel_h_sel = single(uint16(air_wheel(7)) + bitshift(uint16(air_wheel(8)),8)) * single(0.1);
end
status_base = uint8(zeros(8,1));
status_base(1) = active;
status_base(2) = requested;
status_base(3) = uint8(bitand(hin_sel,uint16(255)));
status_base(4) = uint8(bitshift(hin_sel,-8));
status_base(7) = ages(1);
status_base(8) = rx_count(1);
pedal_echo = uint8(zeros(8,1));
pedal_echo(1) = uint8(bitand(ain_sel(1),uint16(255)));
pedal_echo(2) = uint8(bitshift(ain_sel(1),-8));
pedal_echo(3) = uint8(bitand(ain_sel(2),uint16(255)));
pedal_echo(4) = uint8(bitshift(ain_sel(2),-8));
pedal_echo(5) = uint8(bitand(ain_sel(3),uint16(255)));
pedal_echo(6) = uint8(bitshift(ain_sel(3),-8));
if bitand(active,uint8(2)) ~= uint8(0)
    pedal_echo(7) = uint8(1);
end
pedal_echo(8) = rx_count(2);
air_wheel_echo = uint8(zeros(8,1));
air_wheel_echo(1) = uint8(bitand(ain_sel(4),uint16(255)));
air_wheel_echo(2) = uint8(bitshift(ain_sel(4),-8));
air_wheel_echo(3) = uint8(bitand(ain_sel(5),uint16(255)));
air_wheel_echo(4) = uint8(bitshift(ain_sel(5),-8));
wheel_raw = wheel_f_sel * single(10.0);
if wheel_raw <= single(0.0)
    wheel_u16 = uint16(0);
elseif wheel_raw >= single(65535.0)
    wheel_u16 = uint16(65535);
else
    wheel_u16 = uint16(floor(wheel_raw + single(0.5)));
end
air_wheel_echo(5) = uint8(bitand(wheel_u16,uint16(255)));
air_wheel_echo(6) = uint8(bitshift(wheel_u16,-8));
wheel_raw = wheel_h_sel * single(10.0);
if wheel_raw <= single(0.0)
    wheel_u16 = uint16(0);
elseif wheel_raw >= single(65535.0)
    wheel_u16 = uint16(65535);
else
    wheel_u16 = uint16(floor(wheel_raw + single(0.5)));
end
air_wheel_echo(7) = uint8(bitand(wheel_u16,uint16(255)));
air_wheel_echo(8) = uint8(bitshift(wheel_u16,-8));
end

== stateflow chart VCU10/LED_Control/EBS_LED/display ==
  state begin
    spark=T;
  state end
    spark=F;
  (default) -> begin
  begin -> end : after(2,sec)
  data: spark output; T parameter; F parameter
